simulink model "MCity_cs_withAEBSBlock"  (R2017a)
settings: Solver=ode5  StartTime=0.0  StopTime=3.95  FixedStep=1/200  RelTol=1e-3
PreLoadFcn:
  | check_NUTS_defined;
  | 
  | assignin('base',['model_closed_' bdroot],false);
InitFcn:
  | PreScanExperimentInitFcn(bdroot)
StopFcn:
  | PreScanExperimentStopFcn(bdroot)
model workspace (MAT data in the model file):
  mbox_table : struct (value not decoded)
  model_closed = 0
  sim_status = 0
values from neighbouring files (symbols this model uses):
  d_offset = -18.15    [monocityTestLeftTurn.mat]    (also in simulation_leftTurn_PreScan.m = dl/vl*vh - 43 + R)
undefined symbols (not defined in the file or in its folder): DiscIntNeverNeededParam, warningInitialVelocity, x0
libraries: simulink x78, PreScanSimulinkLibrary x14, simulink_extras x10, PreScanUsefulBlocks x4
(part 11 of 12)

== system MCity_cs_withAEBSBlock/BMW_Z3_1/Subsystem/PreBraking Model/Straight road segment/Impact point2 ==
  note: === Impact point block ===
      |
      |    - determines predicted distance to the point of impact,
      |    - passing through zero value, if there is no risk of collision.
  alfa : Inport
  xp [m] : Inport  Port=2
  yp [m] : Inport  Port=3
  Abs : Abs
  Add : Sum  Inputs=+-
  Compare To Constant : simulink/Logic and Bit Operations/Compare To Constant  relop=<  const=-1e-6  OutDataTypeStr=uint8  ZeroCross=off
  Compare To Constant1 : simulink/Logic and Bit Operations/Compare To Constant  relop=>  const=1e-6  OutDataTypeStr=uint8  ZeroCross=off
  Constant : Constant  Value=0
  Divide : Product  Inputs=*/
  Logical Operator : Logic  Operator=OR  AllPortsSameDT=off  OutDataTypeStr=boolean
  Saturation : Saturate  UpperLimit=inf  LowerLimit=1e-6
  Saturation1 : Saturate  UpperLimit=-1e-6  LowerLimit=-inf
  Saturation2 : Saturate  UpperLimit=300  LowerLimit=0
  Switch : Switch  Criteria=u2 > Threshold  Threshold=LaneWidth/2
  Switch1 : Switch  Criteria=u2 > Threshold  Threshold=0.5
  Switch2 : Switch  Criteria=u2 > Threshold
  Trigonometric Function : Trigonometry  Operator=tan
  xp [m]1 : InportShadow  Port=2
  yp [m]1 : InportShadow  Port=3
  xc [m] : Outport
  wires:
  yp [m]/1 -> Abs/1
  xp [m]/1 -> Switch/3
  Constant/1 -> Switch/1
  Switch/1 -> Switch1/3
  Abs/1 -> Switch/2
  xp [m]1/1 -> Add/1
  Divide/1 -> Add/2
  yp [m]1/1 -> Divide/1
  Trigonometric Function/1 -> Divide/2
  alfa/1 -> Compare To Constant1/1, Compare To Constant/1, Saturation1/1, Switch2/2, Saturation/1
  Compare To Constant1/1 -> Logical Operator/1
  Compare To Constant/1 -> Logical Operator/2
  Logical Operator/1 -> Switch1/2
  Switch1/1 -> Saturation2/1
  Add/1 -> Switch1/1
  Switch2/1 -> Trigonometric Function/1
  Saturation/1 -> Switch2/1
  Saturation1/1 -> Switch2/3
  Saturation2/1 -> xc [m]/1

== system MCity_cs_withAEBSBlock/BMW_Z3_1/Subsystem/PreBraking Model/Straight road segment/Relative velocity1 ==
  note: === Relative velocity block ===
      |
      |    - determines:
      |      -- relative, carthesian position of an obstacle,
      |      -- absolute values of carthesian velocity of an obstacle
      |          in respect to the actor orientation,
      |      -- relative velocity Vw beetwen actor and an obstacle
      |          in respect to actor front direction (x).
  V [m/s] : Inport
  range [m] : Inport  Port=2
  rangedot [m/s] : Inport  Port=3
  theta [rad] : Inport  Port=4
  theta_p [rad/s] : Inport  Port=5
  Abs{,1..3} (4 alike) : Abs
  Add : Sum  Inputs=++-
  Add2 : Sum  Inputs=-+
  Constant{,1..3} (4 alike) : Constant  Value=0
  Difference : simulink/Discrete/Difference  ICPrevInput=zeros(TISdet(1),1)  InputProcessing=Inherited  OutMin=[]  OutMax=[]  OutDataType=fixdt(1, 16)  OutScaling=2^-10  DoSatur=off
  Difference1 : simulink/Discrete/Difference  ICPrevInput=zeros(TISdet(1),1)  InputProcessing=Inherited  OutMin=[]  OutMax=[]  OutDataType=fixdt(1, 16)  OutScaling=2^-10  DoSatur=off
  Difference2 : simulink/Discrete/Difference  ICPrevInput=0.0  InputProcessing=Inherited  OutMin=[]  OutMax=[]  OutDataType=sfix(16)  OutScaling=2^-10  DoSatur=off
  Divide : Product  Inputs=**
  Divide1 : Product  Inputs=***
  Divide4 : Product  Inputs=**
  Divide6 : Product  Inputs=**
  Embedded MATLAB Function1 : MATLAB Function  TreatAsAtomicUnit=on
  Gain : Gain  Gain=0.01
  Saturation1 : Saturate  UpperLimit=50  LowerLimit=-50
  Saturation2 : Saturate  UpperLimit=150  LowerLimit=0
  Saturation3 : Saturate  UpperLimit=50  LowerLimit=-50
  Saturation4 : Saturate  UpperLimit=50  LowerLimit=-50
  Saturation5 : Saturate  UpperLimit=11.8  LowerLimit=-11.8
  Switch : Switch  Threshold=0.5
  Switch1 : Switch  Criteria=u2 > Threshold  Threshold=0.8
  Switch2 : Switch  Threshold=10
  Switch3 : Switch  Criteria=u2 > Threshold  Threshold=10
  Translation : MATLAB Function  TreatAsAtomicUnit=on
  Unit Delay : UnitDelay  InitialCondition=zeros(TISdet(1),50)  SampleTime=-1
  cos_theta : Trigonometry  Operator=cos
  sin_theta : Trigonometry
  yp' [m/s] : Outport
  xp' [m/s] : Outport  Port=2
  xp [m] : Outport  Port=3
  yp [m] : Outport  Port=4
  Vw [m/s] : Outport  Port=5
  wires:
  theta [rad]/1 -> cos_theta/1, sin_theta/1
  Divide/1 -> Saturation2/1
  range [m]/1 -> Divide/2, Divide6/1, Divide1/1, Embedded MATLAB Function1/1(r)
  sin_theta/1 -> Divide6/2, Divide1/2
  cos_theta/1 -> Divide/1, Divide4/1
  Divide6/1 -> Saturation5/1
  theta_p [rad/s]/1 -> Divide1/3
  Add2/1 -> Saturation3/1
  Divide4/1 -> Add2/1, Add/2
  Divide1/1 -> Add2/2, Add/3
  Saturation2/1 -> xp [m]/1
  Saturation5/1 -> Embedded MATLAB Function1/2(yp1), yp [m]/1
  Saturation1/1 -> Abs/1, Switch/1
  V [m/s]/1 -> Translation/1(v), Add/1
  Add/1 -> Saturation1/1
  Abs/1 -> Switch/2
  Constant/1 -> Switch/3
  Switch/1 -> Translation/2(xpd)
  Embedded MATLAB Function1/2(K2) -> Unit Delay/1
  Unit Delay/1 -> Embedded MATLAB Function1/3(K1)
  Embedded MATLAB Function1/1(yp2) -> Difference2/1
  Difference2/1 -> Gain/1
  Abs1/1 -> Switch1/2
  Constant1/1 -> Switch1/3
  Saturation4/1 -> yp' [m/s]/1
  Switch1/1 -> Difference/1, Switch2/3
  Switch2/1 -> Saturation4/1
  Difference/1 -> Abs2/1
  Abs2/1 -> Switch2/2
  Translation/1(xp_dot) -> Switch3/3, Difference1/1
  Abs3/1 -> Switch3/2
  Switch3/1 -> xp' [m/s]/1
  Constant2/1 -> Switch2/1
  Constant3/1 -> Switch3/1
  Difference1/1 -> Abs3/1
  rangedot [m/s]/1 -> Divide4/2
  Gain/1 -> Abs1/1, Switch1/1
  Saturation3/1 -> Vw [m/s]/1

== system MCity_cs_withAEBSBlock/BMW_Z3_1/Subsystem/PreBraking Model/Straight road segment/Relative velocity2 ==
  note: === Relative velocity block ===
      |
      |    - determines:
      |      -- relative, carthesian position of an obstacle,
      |      -- absolute values of carthesian velocity of an obstacle
      |          in respect to the actor orientation,
      |      -- relative velocity Vw beetwen actor and an obstacle
      |          in respect to actor front direction (x).
  V [m/s] : Inport
  range [m] : Inport  Port=2
  rangedot [m/s] : Inport  Port=3
  theta [rad] : Inport  Port=4
  theta_p [rad/s] : Inport  Port=5
  Abs{,1..3} (4 alike) : Abs
  Add : Sum  Inputs=++-
  Add2 : Sum  Inputs=-+
  Constant{,1..3} (4 alike) : Constant  Value=0
  Difference : simulink/Discrete/Difference  ICPrevInput=zeros(TISdet(2),1)  InputProcessing=Inherited  OutMin=[]  OutMax=[]  OutDataType=fixdt(1, 16)  OutScaling=2^-10  DoSatur=off
  Difference1 : simulink/Discrete/Difference  ICPrevInput=zeros(TISdet(2),1)  InputProcessing=Inherited  OutMin=[]  OutMax=[]  OutDataType=fixdt(1, 16)  OutScaling=2^-10  DoSatur=off
  Difference2 : simulink/Discrete/Difference  ICPrevInput=0.0  InputProcessing=Inherited  OutMin=[]  OutMax=[]  OutDataType=sfix(16)  OutScaling=2^-10  DoSatur=off
  Divide : Product  Inputs=**
  Divide1 : Product  Inputs=***
  Divide4 : Product  Inputs=**
  Divide6 : Product  Inputs=**
  Embedded MATLAB Function1 : MATLAB Function  TreatAsAtomicUnit=on  SystemSampleTime=0.01
  Gain : Gain  Gain=0.01
  Saturation1 : Saturate  UpperLimit=50  LowerLimit=-50
  Saturation2 : Saturate  UpperLimit=150  LowerLimit=0
  Saturation3 : Saturate  UpperLimit=50  LowerLimit=-50
  Saturation4 : Saturate  UpperLimit=50  LowerLimit=-50
  Saturation5 : Saturate  UpperLimit=11.8  LowerLimit=-11.8
  Switch : Switch  Threshold=0.5
  Switch1 : Switch  Criteria=u2 > Threshold  Threshold=0.8
  Switch2 : Switch  Threshold=10
  Switch3 : Switch  Criteria=u2 > Threshold  Threshold=10
  Translation : MATLAB Function  TreatAsAtomicUnit=on
  Unit Delay : UnitDelay  InitialCondition=zeros(TISdet(2),50)  SampleTime=-1
  cos_theta : Trigonometry  Operator=cos
  sin_theta : Trigonometry
  yp' [m/s] : Outport
  xp' [m/s] : Outport  Port=2
  xp [m] : Outport  Port=3
  yp [m] : Outport  Port=4
  Vw [m/s] : Outport  Port=5
  wires:
  rangedot [m/s]/1 -> Divide4/2
  Difference1/1 -> Abs3/1
  Constant3/1 -> Switch3/1
  Constant2/1 -> Switch2/1
  Switch3/1 -> xp' [m/s]/1
  Abs3/1 -> Switch3/2
  Translation/1(xp_dot) -> Difference1/1, Switch3/3
  Abs2/1 -> Switch2/2
  Difference/1 -> Abs2/1
  Switch2/1 -> Saturation4/1
  Switch1/1 -> Switch2/3, Difference/1
  Saturation4/1 -> yp' [m/s]/1
  Constant1/1 -> Switch1/3
  Abs1/1 -> Switch1/2
  Gain/1 -> Switch1/1, Abs1/1
  Embedded MATLAB Function1/1(yp2) -> Difference2/1
  Unit Delay/1 -> Embedded MATLAB Function1/3(K1)
  Embedded MATLAB Function1/2(K2) -> Unit Delay/1
  Switch/1 -> Translation/2(xpd)
  Constant/1 -> Switch/3
  Abs/1 -> Switch/2
  Add/1 -> Saturation1/1
  V [m/s]/1 -> Translation/1(v), Add/1
  Saturation1/1 -> Switch/1, Abs/1
  Saturation5/1 -> yp [m]/1, Embedded MATLAB Function1/2(yp1)
  Saturation2/1 -> xp [m]/1
  Divide1/1 -> Add/3, Add2/2
  Divide4/1 -> Add/2, Add2/1
  Add2/1 -> Saturation3/1
  theta_p [rad/s]/1 -> Divide1/3
  Divide6/1 -> Saturation5/1
  cos_theta/1 -> Divide/1, Divide4/1
  sin_theta/1 -> Divide6/2, Divide1/2
  range [m]/1 -> Embedded MATLAB Function1/1(r), Divide1/1, Divide6/1, Divide/2
  Divide/1 -> Saturation2/1
  theta [rad]/1 -> cos_theta/1, sin_theta/1
  Difference2/1 -> Gain/1
  Saturation3/1 -> Vw [m/s]/1

== system MCity_cs_withAEBSBlock/BMW_Z3_1/Subsystem/PreBraking Model/Straight road segment/T0.6 ==
  note: === T1.6 block ==
      |
      |    - compare TTC and output adequate binary flag.
  TTC : Inport
  Constant TTC : Inport  Port=2
  Gain : Gain  Gain=2
  Gain2 : Gain  Gain=ones(TISdet(2),1)
  Relational Operator1 : RelationalOperator  Operator=<  OutDataTypeStr=fixdt(1,16)  RndMeth=Nearest
  Switch : Switch  Criteria=u2 > Threshold
  all_flags_0,6 : Outport
  wires:
  Switch/1 -> Relational Operator1/1
  TTC/1 -> Switch/2, Switch/1
  Constant TTC/1 -> Gain2/1
  Gain/1 -> Switch/3
  Gain2/1 -> Gain/1, Relational Operator1/2
  Relational Operator1/1 -> all_flags_0,6/1

== system MCity_cs_withAEBSBlock/BMW_Z3_1/Subsystem/PreBraking Model/Straight road segment/T1.6 ==
  note: === T1.6 block ==
      |
      |    - compare TTC and output adequate binary flag.
  TTC : Inport
  Constant TTC : Inport  Port=2
  Gain : Gain  Gain=2
  Gain2 : Gain  Gain=ones(TISdet(1),1)
  Relational Operator1 : RelationalOperator  Operator=<  OutDataTypeStr=fixdt(1,16)  RndMeth=Nearest
  Switch : Switch  Criteria=u2 > Threshold
  median filter : Subsystem
  all_flags_1.6 : Outport
  wires:
  Switch/1 -> Relational Operator1/1
  Relational Operator1/1 -> median filter/1(Flag in)
  TTC/1 -> Switch/2, Switch/1
  Constant TTC/1 -> Gain2/1
  Gain/1 -> Switch/3
  Gain2/1 -> Gain/1, Relational Operator1/2
  median filter/1(Flag out) -> all_flags_1.6/1

== system MCity_cs_withAEBSBlock/BMW_Z3_1/Subsystem/PreBraking Model/Straight road segment/T2.6 ==
  note: === T1.6 block ==
      |
      |    - compare TTC and output adequate binary flag.
  TTC : Inport
  Constant TTC : Inport  Port=2
  Gain : Gain  Gain=2
  Gain2 : Gain  Gain=ones(TISdet(1),1)
  Relational Operator1 : RelationalOperator  Operator=<  OutDataTypeStr=fixdt(1,16)  RndMeth=Nearest
  Switch : Switch  Criteria=u2 > Threshold
  median filter : Subsystem
  all_flags_2.6 : Outport
  wires:
  Switch/1 -> Relational Operator1/1
  TTC/1 -> Switch/2, Switch/1
  Constant TTC/1 -> Gain2/1
  Gain/1 -> Switch/3
  Gain2/1 -> Gain/1, Relational Operator1/2
  Relational Operator1/1 -> median filter/1(Flag in)
  median filter/1(Flag out) -> all_flags_2.6/1

== system MCity_cs_withAEBSBlock/BMW_Z3_1/Subsystem/PreBraking Model/Straight road segment/THETA Derivative1 ==
  note: === Theta derivative block ===
      |
      |    - computs derivative of the theta using linear
      |       extrapolation and correction method
  range [m] : Inport
  theta [rad] : Inport  Port=2
  Abs1 : Abs
  Deriv correction : MATLAB Function  TreatAsAtomicUnit=on
  Difference1 : simulink/Discrete/Difference  ICPrevInput=0.0  InputProcessing=Inherited  OutMin=[]  OutMax=[]  OutDataType=sfix(16)  OutScaling=2^-10  DoSatur=off
  Difference2 : simulink/Discrete/Difference  ICPrevInput=0.0  InputProcessing=Inherited  OutMin=[]  OutMax=[]  OutDataType=sfix(16)  OutScaling=2^-10  DoSatur=off
  Digital Clock : DigitalClock  SampleTime=min(Tsensor)
  Gain : Gain  Gain=Tsensor(2)
  Gain1 : Gain  Gain=Tsensor(2)
  Switch : Switch  Threshold=2
  Theta extrapolation : MATLAB Function  TreatAsAtomicUnit=on
  Unit Delay : UnitDelay  InitialCondition=zeros(TISdet(2),1)  SampleTime=-1
  Unit Delay1 : UnitDelay  InitialCondition=zeros(TISdet(2),10,2)  SampleTime=-1
  Unit Delay2 : UnitDelay  InitialCondition=zeros(TISdet(2),1)  SampleTime=-1
  theta_dot [rad/s] : Outport
  wires:
  Unit Delay2/1 -> Deriv correction/2(thp)
  Gain1/1 -> Deriv correction/3(thd)
  Theta extrapolation/1(th2) -> Deriv correction/1(th), Unit Delay2/1, Difference1/1
  range [m]/1 -> Theta extrapolation/1(r)
  Gain/1 -> Theta extrapolation/3(thd)
  Digital Clock/1 -> Theta extrapolation/4(time)
  Unit Delay1/1 -> Theta extrapolation/5(K1)
  Theta extrapolation/2(K2) -> Unit Delay1/1
  theta [rad]/1 -> Theta extrapolation/2(th1), Difference2/1
  Deriv correction/1(th_dot) -> Switch/3, Abs1/1
  Switch/1 -> theta_dot [rad/s]/1, Unit Delay/1
  Abs1/1 -> Switch/2
  Unit Delay/1 -> Switch/1
  Difference2/1 -> Gain/1
  Difference1/1 -> Gain1/1

== system MCity_cs_withAEBSBlock/BMW_Z3_1/Subsystem/PreBraking Model/Straight road segment/THETA Derivative2 ==
  note: === Theta derivative block ===
      |
      |    - computs derivative of the theta using linear
      |       extrapolation and correction method
  range [m] : Inport
  theta [rad] : Inport  Port=2
  Abs1 : Abs
  Deriv correction : MATLAB Function  TreatAsAtomicUnit=on
  Difference1 : simulink/Discrete/Difference  ICPrevInput=0.0  InputProcessing=Inherited  OutMin=[]  OutMax=[]  OutDataType=sfix(16)  OutScaling=2^-10  DoSatur=off
  Difference2 : simulink/Discrete/Difference  ICPrevInput=0.0  InputProcessing=Inherited  OutMin=[]  OutMax=[]  OutDataType=sfix(16)  OutScaling=2^-10  DoSatur=off
  Digital Clock : DigitalClock  SampleTime=min(Tsensor)
  Gain : Gain  Gain=Tsensor(1)
  Gain1 : Gain  Gain=Tsensor(1)
  Switch : Switch  Threshold=2
  Theta extrapolation : MATLAB Function  TreatAsAtomicUnit=on
  Unit Delay : UnitDelay  InitialCondition=zeros(TISdet(1),1)  SampleTime=-1
  Unit Delay1 : UnitDelay  InitialCondition=zeros(TISdet(1),10,2)  SampleTime=-1
  Unit Delay2 : UnitDelay  InitialCondition=zeros(TISdet(1),1)  SampleTime=-1
  theta_dot [rad/s] : Outport
  wires:
  Unit Delay2/1 -> Deriv correction/2(thp)
  Gain1/1 -> Deriv correction/3(thd)
  Theta extrapolation/1(th2) -> Deriv correction/1(th), Unit Delay2/1, Difference1/1
  range [m]/1 -> Theta extrapolation/1(r)
  Gain/1 -> Theta extrapolation/3(thd)
  Digital Clock/1 -> Theta extrapolation/4(time)
  Unit Delay1/1 -> Theta extrapolation/5(K1)
  Theta extrapolation/2(K2) -> Unit Delay1/1
  theta [rad]/1 -> Theta extrapolation/2(th1), Difference2/1
  Deriv correction/1(th_dot) -> Switch/3, Abs1/1
  Switch/1 -> theta_dot [rad/s]/1, Unit Delay/1
  Abs1/1 -> Switch/2
  Unit Delay/1 -> Switch/1
  Difference2/1 -> Gain/1
  Difference1/1 -> Gain1/1

== system MCity_cs_withAEBSBlock/BMW_Z3_1/Subsystem/PreBraking Model/Straight road segment/TTC computing ==
  xc [m] : Inport
  Vw [m/s] : Inport  Port=2
  Compare To Constant : simulink/Logic and Bit Operations/Compare To Constant  relop===  const=1e-6  OutDataTypeStr=uint8  ZeroCross=off
  Constant : Constant  Value=0
  Data Type Conversion : DataTypeConversion
  Divide : Product  Inputs=/*
  Saturation : Saturate  UpperLimit=inf  LowerLimit=1e-6
  Switch : Switch  Criteria=u2 > Threshold
  Switch1 : Switch  Criteria=u2 > Threshold  Threshold=0.5
  TTC : Outport  InitialOutput=0
  wires:
  Vw [m/s]/1 -> Switch/2, Switch/1
  Constant/1 -> Switch1/1, Switch/3
  Switch/1 -> Saturation/1
  Saturation/1 -> Divide/1, Compare To Constant/1
  Compare To Constant/1 -> Data Type Conversion/1
  xc [m]/1 -> Divide/2
  Divide/1 -> Switch1/3
  Switch1/1 -> TTC/1
  Data Type Conversion/1 -> Switch1/2

== system MCity_cs_withAEBSBlock/BMW_Z3_1/Subsystem/PreBraking Model/Straight road segment/TTC computing1 ==
  xc [m] : Inport
  Vw [m/s] : Inport  Port=2
  Compare To Constant : simulink/Logic and Bit Operations/Compare To Constant  relop===  const=1e-6  OutDataTypeStr=uint8  ZeroCross=off
  Constant : Constant  Value=0
  Data Type Conversion : DataTypeConversion
  Divide : Product  Inputs=/*
  Saturation : Saturate  UpperLimit=inf  LowerLimit=1e-6
  Switch : Switch  Criteria=u2 > Threshold
  Switch1 : Switch  Criteria=u2 > Threshold  Threshold=0.5
  TTC : Outport  InitialOutput=0
  wires:
  Vw [m/s]/1 -> Switch/2, Switch/1
  Constant/1 -> Switch/3, Switch1/1
  Switch/1 -> Saturation/1
  Saturation/1 -> Divide/1, Compare To Constant/1
  Compare To Constant/1 -> Data Type Conversion/1
  xc [m]/1 -> Divide/2
  Divide/1 -> Switch1/3
  Switch1/1 -> TTC/1
  Data Type Conversion/1 -> Switch1/2

== system MCity_cs_withAEBSBlock/BMW_Z3_1/Subsystem/PreBraking Model/Straight road segment/alfa ==
  yp'1 : Inport
  xp' : Inport  Port=2
  Abs : Abs
  Compare To Constant : simulink/Logic and Bit Operations/Compare To Constant  relop===  const=pi/2  OutDataTypeStr=uint8
  Constant : Constant  Value=0
  Switch : Switch  Criteria=u2 > Threshold
  four quadrant atan : Trigonometry  Operator=atan2
  alfa1 : Outport
  wires:
  yp'1/1 -> four quadrant atan/1
  xp'/1 -> four quadrant atan/2
  four quadrant atan/1 -> Abs/1, Switch/3
  Abs/1 -> Compare To Constant/1
  Compare To Constant/1 -> Switch/2
  Constant/1 -> Switch/1
  Switch/1 -> alfa1/1

== system MCity_cs_withAEBSBlock/BMW_Z3_1/Subsystem/PreBraking Model/Straight road segment/alfa1 ==
  yp'1 : Inport
  xp' : Inport  Port=2
  Abs : Abs
  Compare To Constant : simulink/Logic and Bit Operations/Compare To Constant  relop===  const=pi/2  OutDataTypeStr=uint8
  Constant : Constant  Value=0
  Switch : Switch  Criteria=u2 > Threshold
  four quadrant atan : Trigonometry  Operator=atan2
  alfa1 : Outport
  wires:
  yp'1/1 -> four quadrant atan/1
  xp'/1 -> four quadrant atan/2
  four quadrant atan/1 -> Abs/1, Switch/3
  Abs/1 -> Compare To Constant/1
  Compare To Constant/1 -> Switch/2
  Constant/1 -> Switch/1
  Switch/1 -> alfa1/1

== system MCity_cs_withAEBSBlock/BMW_Z3_1/Trajectories/Traj2State1/Traj2State2/MuxState ==
  x [m] : Inport
  y [m] : Inport  Port=2
  z [m] : Inport  Port=3
  dx [m/s] : Inport  Port=4
  dy [m/s] : Inport  Port=5
  dz [m/s] : Inport  Port=6
  R [rad] : Inport  Port=7
  P [rad] : Inport  Port=8
  Y [rad] : Inport  Port=9
  Mux : Mux  Inputs=9
  state : Outport
  wires:
  z [m]/1 -> Mux/3
  y [m]/1 -> Mux/2
  x [m]/1 -> Mux/1
  Y [rad]/1 -> Mux/9
  P [rad]/1 -> Mux/8
  R [rad]/1 -> Mux/7
  dz [m/s]/1 -> Mux/6
  dy [m/s]/1 -> Mux/5
  dx [m/s]/1 -> Mux/4
  Mux/1 -> state/1

== system MCity_cs_withAEBSBlock/BMW_Z3_1/Trajectories/Traj2State1/Traj2State2/Traj2MuxState_Ext ==
  Traj : Inport
  Terminator{1..9} (9 alike) : Terminator
  demux : Subsystem
  x [m] : Outport
  y [m] : Outport  Port=2
  z [m] : Outport  Port=3
  dx [m/s] : Outport  Port=4
  dy [m/s] : Outport  Port=5
  dz [m/s] : Outport  Port=6
  R [rad] : Outport  Port=7
  P [rad] : Outport  Port=8
  Y [rad] : Outport  Port=9
  wires:
  demux/9(Y) -> Y [rad]/1
  demux/7(R) -> R [rad]/1
  demux/5(vely) -> dy [m/s]/1
  demux/4(velx) -> dx [m/s]/1
  demux/10(velR) -> Terminator4/1
  demux/11(velP) -> Terminator5/1
  demux/12(velY) -> Terminator1/1
  demux/13(accx) -> Terminator8/1
  demux/14(accy) -> Terminator9/1
  demux/15(accz) -> Terminator7/1
  demux/18(accY) -> Terminator2/1
  demux/16(accR) -> Terminator3/1
  demux/17(accP) -> Terminator6/1
  demux/3(z) -> z [m]/1
  Traj/1 -> demux/1(traj)
  demux/6(velz) -> dz [m/s]/1
  demux/1(x) -> x [m]/1
  demux/2(y) -> y [m]/1
  demux/8(P) -> P [rad]/1

== system MCity_cs_withAEBSBlock/Audi_A8_1/Dynamics_Simple/Chassis/Bicycle_model_[XYZ]/X_Motion/Air&RoadResistance ==
  vx_[ms-1] : Inport
  Gain : Gain  Gain=1/p.Rw
  Road & Aerodyn Resistances : Fcn  Expr=p.Rroad + p.Rair*u^2
  Saturation1 : Saturate  UpperLimit=5/15  LowerLimit=-5/15
  Sign : Signum
  "[ms-1] 2 [rads-1]" : Gain  Gain=1/p.Rw  SaturateOnIntegerOverflow=on  OutDataTypeStr=Inherit: Same as input  ParamDataTypeStr=Inherit: Same as input
  signed load1 : Product  SaturateOnIntegerOverflow=on  InputSameDT=on  OutDataTypeStr=Inherit: Same as first input
  Resistance_Force : Outport
  wires:
  signed load1/1 -> Resistance_Force/1  "F_[N]"
  vx_[ms-1]/1 -> Road & Aerodyn Resistances/1, "[ms-1] 2 [rads-1]"/1
  Saturation1/1 -> Sign/1
  "[ms-1] 2 [rads-1]"/1 -> Saturation1/1
  Road & Aerodyn Resistances/1 -> Gain/1  "ResistanceTorque_[Nm]"
  Sign/1 -> signed load1/2  "sign"
  Gain/1 -> signed load1/1  "Resistance Force_[N]"

== system MCity_cs_withAEBSBlock/Audi_A8_1/Dynamics_Simple/Chassis/Bicycle_model_[XYZ]/X_Motion/BrakeSystem ==
  vx_[ms-1] : Inport
  BrakePressure_[bar] : Inport  Port=2
  Gain : Gain  Gain=1/p.Rw
  Saturation : Saturate  UpperLimit=p.PBrakeMax  LowerLimit=0
  Saturation1 : Saturate  UpperLimit=5/15  LowerLimit=-5/15
  Sign : Signum
  "[ms-1] 2 [rads-1]" : Gain  Gain=1/p.Rw  SaturateOnIntegerOverflow=on  OutDataTypeStr=Inherit: Same as input  ParamDataTypeStr=Inherit: Same as input
  braking Q factor : Gain  Gain=p.Qfac  SaturateOnIntegerOverflow=on  OutDataTypeStr=Inherit: Same as input  ParamDataTypeStr=Inherit: Same as input
  signed load1 : Product  SaturateOnIntegerOverflow=on  InputSameDT=on  OutDataTypeStr=Inherit: Same as first input
  BrakeForce : Outport
  BrakeTorqueAbs : Outport  Port=2
  wires:
  braking Q factor/1 -> BrakeTorqueAbs/1, Gain/1
  BrakePressure_[bar]/1 -> Saturation/1
  Saturation/1 -> braking Q factor/1
  vx_[ms-1]/1 -> "[ms-1] 2 [rads-1]"/1
  Saturation1/1 -> Sign/1
  "[ms-1] 2 [rads-1]"/1 -> Saturation1/1
  Sign/1 -> signed load1/2  "sign"
  signed load1/1 -> BrakeForce/1
  Gain/1 -> signed load1/1

== system MCity_cs_withAEBSBlock/Audi_A8_1/Dynamics_Simple/Chassis/Bicycle_model_[XYZ]/X_Motion/Configurable Subsystem ==
  In1 : Inport
  In2 : Inport  Port=2
  In3 : Inport  Port=3
  Integrator : Integrator  ExternalReset=level  InitialConditionSource=external
  Out1 : Outport
  wires:
  In1/1 -> Integrator/1
  In2/1 -> Integrator/2
  In3/1 -> Integrator/3
  Integrator/1 -> Out1/1

== system MCity_cs_withAEBSBlock/Audi_A8_1/Dynamics_Simple/Chassis/Bicycle_model_[XYZ]/X_Motion/Configurable Subsystem1 ==
  In1 : Inport
  Torsional damping : TransferFcn  Denominator=[0.1 1]
  Out1 : Outport
  wires:
  In1/1 -> Torsional damping/1
  Torsional damping/1 -> Out1/1

== system MCity_cs_withAEBSBlock/Audi_A8_1/Dynamics_Simple/Chassis/Bicycle_model_[XYZ]/X_Motion/Max RPM and zero- velocity detection ==
  note: Set to zero after infinite small time-step
  note: Zero velocity detection
  ax : Inport
  Drive Torque : Inport  Port=2
  Brake Torque : Inport  Port=3
  v0 : Inport  Port=4
  vx : Inport  Port=5
  Abs : Abs
  Abs1 : Abs
  Compare To Zero : simulink/Logic and Bit Operations/Compare To Zero  relop=<=  OutDataTypeStr=boolean  ZeroCross=off
  Compare To Zero1 : simulink/Logic and Bit Operations/Compare To Zero  relop=>=  OutDataTypeStr=boolean  ZeroCross=off
  Compare To Zero2 : simulink/Logic and Bit Operations/Compare To Zero  relop=>=  OutDataTypeStr=boolean  ZeroCross=off
  Compare To Zero3 : simulink/Logic and Bit Operations/Compare To Zero  relop=<=  OutDataTypeStr=boolean  ZeroCross=off
  Configurable Subsystem : Subsystem  BlockChoice=Step  mask{ComputationMode=ComputationMode}
      mask prompts: ComputationMode "Compuation mode:"
      mask init:
      | SetComputationMode(gcb,ComputationMode);
      settings: AttributesFormatString=%<BlockChoice>  OpenFcn=BringToFront(gcb);  MemberBlocks=Discrete Step,Step
      settings: TemplateBlock=|
      | PreScanSimulinkLibrary/Configurable Subsystems/Step Function/Configurable
      | Subsystem
  Constant : Constant
  Constant1 : Constant
  Logical Operator : Logic  AllPortsSameDT=off  OutDataTypeStr=boolean
  Logical Operator1 : Logic  AllPortsSameDT=off  OutDataTypeStr=boolean
  Logical Operator2 : Logic  Operator=NOT  AllPortsSameDT=off  OutDataTypeStr=boolean
  Logical Operator3 : Logic  AllPortsSameDT=off  OutDataTypeStr=boolean
  Logical Operator4 : Logic  Operator=OR  AllPortsSameDT=off  OutDataTypeStr=boolean
  Memory : Memory
  Memory1 : Memory
  Memory2 : Memory
  Product : Product  RndMeth=Zero
  Relational Operator : RelationalOperator  Operator=<  OutDataTypeStr=boolean  RndMeth=Nearest
  SR-Memory : Subsystem
  Sum : Sum  Inputs=|-+
  Switch : Switch  Criteria=u2 ~= 0  Threshold=0.5
  ax is 0 : Constant  Value=0
  ax_out : Outport
  vx_reset : Outport  Port=2
  x0 : Outport  Port=3
  wires:
  Logical Operator4/1 -> Logical Operator1/1
  vx/1 -> Compare To Zero/1, Compare To Zero2/1, Memory2/1, Memory/1  "vx"
  Memory2/1 -> Compare To Zero3/1
  Compare To Zero2/1 -> Logical Operator3/1
  Compare To Zero3/1 -> Logical Operator3/2
  Logical Operator3/1 -> Logical Operator4/2  "zero-crossing backward"
  Memory/1 -> Compare To Zero1/1
  Compare To Zero/1 -> Logical Operator/1
  Compare To Zero1/1 -> Logical Operator/2
  Logical Operator/1 -> Logical Operator4/1  "zero-crossing forward"
  Abs/1 -> Relational Operator/1
  Abs1/1 -> Relational Operator/2
  Drive Torque/1 -> Abs/1
  Brake Torque/1 -> Abs1/1
  Relational Operator/1 -> Logical Operator1/2, Logical Operator2/1
  Logical Operator1/1 -> SR-Memory/2(Set)
  Constant/1 -> SR-Memory/1(Signal)
  Logical Operator2/1 -> SR-Memory/3(Reset)
  SR-Memory/1(Out) -> Sum/1, Memory1/1
  Switch/1 -> ax_out/1
  Sum/1 -> Switch/2
  ax is 0/1 -> Switch/3
  Constant1/1 -> Sum/2
  v0/1 -> Product/1
  Product/1 -> x0/1
  Configurable Subsystem/1(Out1) -> Product/2
  ax/1 -> Switch/1  "ax"
  Memory1/1 -> vx_reset/1  "vx"

== system MCity_cs_withAEBSBlock/Audi_A8_1/Dynamics_Simple/Chassis/Bicycle_model_[XYZ]/Y & Yaw_Motion/Configurable Subsystem ==
  In1 : Inport
  In2 : Inport  Port=2
  Integrator : Integrator  ExternalReset=level
  Out1 : Outport
  wires:
  In1/1 -> Integrator/1
  In2/1 -> Integrator/2
  Integrator/1 -> Out1/1

== system MCity_cs_withAEBSBlock/Audi_A8_1/Dynamics_Simple/Chassis/Bicycle_model_[XYZ]/Y & Yaw_Motion/Configurable Subsystem1 ==
  In1 : Inport
  Integrator : Integrator
  Out1 : Outport
  wires:
  In1/1 -> Integrator/1
  Integrator/1 -> Out1/1

== system MCity_cs_withAEBSBlock/Audi_A8_1/Dynamics_Simple/Chassis/Bicycle_model_[XYZ]/Y & Yaw_Motion/Configurable Subsystem2 ==
  In1 : Inport
  In2 : Inport  Port=2
  Integrator : Integrator  ExternalReset=level
  Out1 : Outport
  wires:
  In1/1 -> Integrator/1
  In2/1 -> Integrator/2
  Integrator/1 -> Out1/1

== system MCity_cs_withAEBSBlock/Audi_A8_1/Dynamics_Simple/Chassis/Bicycle_model_[XYZ]/Z, Pitch_Motion & Roll_Motion/Configurable Subsystem ==
  In1 : Inport
  Integrator : Integrator  LimitOutput=on  UpperSaturationLimit=5*pi/180  LowerSaturationLimit=-5*pi/180
  Out1 : Outport
  wires:
  In1/1 -> Integrator/1
  Integrator/1 -> Out1/1

== system MCity_cs_withAEBSBlock/Audi_A8_1/Dynamics_Simple/Chassis/Bicycle_model_[XYZ]/Z, Pitch_Motion & Roll_Motion/Configurable Subsystem1 ==
  In1 : Inport
  Integrator : Integrator
  Out1 : Outport
  wires:
  In1/1 -> Integrator/1
  Integrator/1 -> Out1/1

== system MCity_cs_withAEBSBlock/Audi_A8_1/Dynamics_Simple/Chassis/Bicycle_model_[XYZ]/Z, Pitch_Motion & Roll_Motion/Configurable Subsystem2 ==
  In1 : Inport
  Integrator : Integrator
  Out1 : Outport
  wires:
  In1/1 -> Integrator/1
  Integrator/1 -> Out1/1

== system MCity_cs_withAEBSBlock/Audi_A8_1/Dynamics_Simple/Chassis/Bicycle_model_[XYZ]/Z, Pitch_Motion & Roll_Motion/Configurable Subsystem3 ==
  In1 : Inport
  Integrator : Integrator
  Out1 : Outport
  wires:
  In1/1 -> Integrator/1
  Integrator/1 -> Out1/1

== system MCity_cs_withAEBSBlock/Audi_A8_1/Dynamics_Simple/Chassis/Bicycle_model_[XYZ]/Z, Pitch_Motion & Roll_Motion/Configurable Subsystem4 ==
  In1 : Inport
  Integrator : Integrator
  Out1 : Outport
  wires:
  In1/1 -> Integrator/1
  Integrator/1 -> Out1/1

== system MCity_cs_withAEBSBlock/Audi_A8_1/Dynamics_Simple/Chassis/Bicycle_model_[XYZ]/Z, Pitch_Motion & Roll_Motion/Configurable Subsystem5 ==
  In1 : Inport
  Integrator : Integrator
  Out1 : Outport
  wires:
  In1/1 -> Integrator/1
  Integrator/1 -> Out1/1

== system MCity_cs_withAEBSBlock/Audi_A8_1/Dynamics_Simple/Chassis/Bicycle_model_[XYZ]/Z, Pitch_Motion & Roll_Motion/Configurable Subsystem9 ==
  In1 : Inport
  Derivative : Derivative
  Out1 : Outport
  wires:
  In1/1 -> Derivative/1
  Derivative/1 -> Out1/1

== system MCity_cs_withAEBSBlock/Audi_A8_1/Dynamics_Simple/Chassis/FrontTyre/AlphaFront/Enabled Subsystem ==
  In : Inport
  Enable : EnablePort  PropagateVarSize=During execution
  AlphaFront : Fcn  Expr=-atan( (u(2)+u(3)*p.a)/u(1) )
  Alpha : Outport  OutputWhenDisabled=reset  InitialOutput=[0]
  wires:
  AlphaFront/1 -> Alpha/1
  In/1 -> AlphaFront/1

== system MCity_cs_withAEBSBlock/Audi_A8_1/Dynamics_Simple/Chassis/RearTyre/AlphaRear/Enabled Subsystem ==
  In : Inport
  Enable : EnablePort  PropagateVarSize=During execution
  AlphaRear : Fcn  Expr=-atan( (u(2)-u(3)*p.b)/u(1) )
  Alpha : Outport  OutputWhenDisabled=reset  InitialOutput=[0]
  wires:
  AlphaRear/1 -> Alpha/1
  In/1 -> AlphaRear/1

== system MCity_cs_withAEBSBlock/Audi_A8_1/Trajectories/Traj2State1/Traj2State2/Traj2MuxState_Ext/demux ==
  traj : Inport
  Demux : Demux  Outputs=18
  x : Outport
  y : Outport  Port=2
  z : Outport  Port=3
  velx : Outport  Port=4
  vely : Outport  Port=5
  velz : Outport  Port=6
  R : Outport  Port=7
  P : Outport  Port=8
  Y : Outport  Port=9
  velR : Outport  Port=10
  velP : Outport  Port=11
  velY : Outport  Port=12
  accx : Outport  Port=13
  accy : Outport  Port=14
  accz : Outport  Port=15
  accR : Outport  Port=16
  accP : Outport  Port=17
  accY : Outport  Port=18
  wires:
  Demux/18 -> accY/1
  Demux/17 -> accP/1
  Demux/16 -> accR/1
  Demux/15 -> accz/1
  Demux/14 -> accy/1
  Demux/13 -> accx/1
  Demux/12 -> velY/1
  Demux/11 -> velP/1
  Demux/10 -> velR/1
  Demux/9 -> velz/1
  Demux/8 -> vely/1
  Demux/7 -> velx/1
  Demux/6 -> Y/1
  Demux/5 -> P/1
  traj/1 -> Demux/1
  Demux/4 -> R/1
  Demux/3 -> z/1
  Demux/2 -> y/1
  Demux/1 -> x/1

== system MCity_cs_withAEBSBlock/BMW_Z3_1/Dynamics_Simple/Chassis/Bicycle_model_[XYZ]/X_Motion/Air&RoadResistance ==
  vx_[ms-1] : Inport
  Gain : Gain  Gain=1/p.Rw
  Road & Aerodyn Resistances : Fcn  Expr=p.Rroad + p.Rair*u^2
  Saturation1 : Saturate  UpperLimit=5/15  LowerLimit=-5/15
  Sign : Signum
  "[ms-1] 2 [rads-1]" : Gain  Gain=1/p.Rw  SaturateOnIntegerOverflow=on  OutDataTypeStr=Inherit: Same as input  ParamDataTypeStr=Inherit: Same as input
  signed load1 : Product  SaturateOnIntegerOverflow=on  InputSameDT=on  OutDataTypeStr=Inherit: Same as first input
  Resistance_Force : Outport
  wires:
  signed load1/1 -> Resistance_Force/1  "F_[N]"
  vx_[ms-1]/1 -> Road & Aerodyn Resistances/1, "[ms-1] 2 [rads-1]"/1
  Saturation1/1 -> Sign/1
  "[ms-1] 2 [rads-1]"/1 -> Saturation1/1
  Road & Aerodyn Resistances/1 -> Gain/1  "ResistanceTorque_[Nm]"
  Sign/1 -> signed load1/2  "sign"
  Gain/1 -> signed load1/1  "Resistance Force_[N]"

== system MCity_cs_withAEBSBlock/BMW_Z3_1/Dynamics_Simple/Chassis/Bicycle_model_[XYZ]/X_Motion/BrakeSystem ==
  vx_[ms-1] : Inport
  BrakePressure_[bar] : Inport  Port=2
  Gain : Gain  Gain=1/p.Rw
  Saturation : Saturate  UpperLimit=p.PBrakeMax  LowerLimit=0
  Saturation1 : Saturate  UpperLimit=5/15  LowerLimit=-5/15
  Sign : Signum
  "[ms-1] 2 [rads-1]" : Gain  Gain=1/p.Rw  SaturateOnIntegerOverflow=on  OutDataTypeStr=Inherit: Same as input  ParamDataTypeStr=Inherit: Same as input
  braking Q factor : Gain  Gain=p.Qfac  SaturateOnIntegerOverflow=on  OutDataTypeStr=Inherit: Same as input  ParamDataTypeStr=Inherit: Same as input
  signed load1 : Product  SaturateOnIntegerOverflow=on  InputSameDT=on  OutDataTypeStr=Inherit: Same as first input
  BrakeForce : Outport
  BrakeTorqueAbs : Outport  Port=2
  wires:
  braking Q factor/1 -> BrakeTorqueAbs/1, Gain/1
  BrakePressure_[bar]/1 -> Saturation/1
  Saturation/1 -> braking Q factor/1
  vx_[ms-1]/1 -> "[ms-1] 2 [rads-1]"/1
  Saturation1/1 -> Sign/1
  "[ms-1] 2 [rads-1]"/1 -> Saturation1/1
  Sign/1 -> signed load1/2  "sign"
  signed load1/1 -> BrakeForce/1
  Gain/1 -> signed load1/1

== system MCity_cs_withAEBSBlock/BMW_Z3_1/Dynamics_Simple/Chassis/Bicycle_model_[XYZ]/X_Motion/Configurable Subsystem ==
  In1 : Inport
  In2 : Inport  Port=2
  In3 : Inport  Port=3
  Integrator : Integrator  ExternalReset=level  InitialConditionSource=external
  Out1 : Outport
  wires:
  In1/1 -> Integrator/1
  In2/1 -> Integrator/2
  In3/1 -> Integrator/3
  Integrator/1 -> Out1/1

== system MCity_cs_withAEBSBlock/BMW_Z3_1/Dynamics_Simple/Chassis/Bicycle_model_[XYZ]/X_Motion/Configurable Subsystem1 ==
  In1 : Inport
  Torsional damping : TransferFcn  Denominator=[0.1 1]
  Out1 : Outport
  wires:
  In1/1 -> Torsional damping/1
  Torsional damping/1 -> Out1/1

== system MCity_cs_withAEBSBlock/BMW_Z3_1/Dynamics_Simple/Chassis/Bicycle_model_[XYZ]/X_Motion/Max RPM and zero- velocity detection ==
  note: Set to zero after infinite small time-step
  note: Zero velocity detection
  ax : Inport
  Drive Torque : Inport  Port=2
  Brake Torque : Inport  Port=3
  v0 : Inport  Port=4
  vx : Inport  Port=5
  Abs : Abs
  Abs1 : Abs
  Compare To Zero : simulink/Logic and Bit Operations/Compare To Zero  relop=<=  OutDataTypeStr=boolean  ZeroCross=off
  Compare To Zero1 : simulink/Logic and Bit Operations/Compare To Zero  relop=>=  OutDataTypeStr=boolean  ZeroCross=off
  Compare To Zero2 : simulink/Logic and Bit Operations/Compare To Zero  relop=>=  OutDataTypeStr=boolean  ZeroCross=off
  Compare To Zero3 : simulink/Logic and Bit Operations/Compare To Zero  relop=<=  OutDataTypeStr=boolean  ZeroCross=off
  Configurable Subsystem : Subsystem  BlockChoice=Step  mask{ComputationMode=ComputationMode}
      mask prompts: ComputationMode "Compuation mode:"
      mask init:
      | SetComputationMode(gcb,ComputationMode);
      settings: AttributesFormatString=%<BlockChoice>  OpenFcn=BringToFront(gcb);  MemberBlocks=Discrete Step,Step
      settings: TemplateBlock=|
      | PreScanSimulinkLibrary/Configurable Subsystems/Step Function/Configurable
      | Subsystem
  Constant : Constant
  Constant1 : Constant
  Logical Operator : Logic  AllPortsSameDT=off  OutDataTypeStr=boolean
  Logical Operator1 : Logic  AllPortsSameDT=off  OutDataTypeStr=boolean
  Logical Operator2 : Logic  Operator=NOT  AllPortsSameDT=off  OutDataTypeStr=boolean
  Logical Operator3 : Logic  AllPortsSameDT=off  OutDataTypeStr=boolean
  Logical Operator4 : Logic  Operator=OR  AllPortsSameDT=off  OutDataTypeStr=boolean
  Memory : Memory
  Memory1 : Memory
  Memory2 : Memory
  Product : Product  RndMeth=Zero
  Relational Operator : RelationalOperator  Operator=<  OutDataTypeStr=boolean  RndMeth=Nearest
  SR-Memory : Subsystem
  Sum : Sum  Inputs=|-+
  Switch : Switch  Criteria=u2 ~= 0  Threshold=0.5
  ax is 0 : Constant  Value=0
  ax_out : Outport
  vx_reset : Outport  Port=2
  x0 : Outport  Port=3
  wires:
  Logical Operator4/1 -> Logical Operator1/1
  vx/1 -> Compare To Zero/1, Compare To Zero2/1, Memory2/1, Memory/1  "vx"
  Memory2/1 -> Compare To Zero3/1
  Compare To Zero2/1 -> Logical Operator3/1
  Compare To Zero3/1 -> Logical Operator3/2
  Logical Operator3/1 -> Logical Operator4/2  "zero-crossing backward"
  Memory/1 -> Compare To Zero1/1
  Compare To Zero/1 -> Logical Operator/1
  Compare To Zero1/1 -> Logical Operator/2
  Logical Operator/1 -> Logical Operator4/1  "zero-crossing forward"
  Abs/1 -> Relational Operator/1
  Abs1/1 -> Relational Operator/2
  Drive Torque/1 -> Abs/1
  Brake Torque/1 -> Abs1/1
  Relational Operator/1 -> Logical Operator1/2, Logical Operator2/1
  Logical Operator1/1 -> SR-Memory/2(Set)
  Constant/1 -> SR-Memory/1(Signal)
  Logical Operator2/1 -> SR-Memory/3(Reset)
  SR-Memory/1(Out) -> Sum/1, Memory1/1
  Switch/1 -> ax_out/1
  Sum/1 -> Switch/2
  ax is 0/1 -> Switch/3
  Constant1/1 -> Sum/2
  v0/1 -> Product/1
  Product/1 -> x0/1
  Configurable Subsystem/1(Out1) -> Product/2
  ax/1 -> Switch/1  "ax"
  Memory1/1 -> vx_reset/1  "vx"

== system MCity_cs_withAEBSBlock/BMW_Z3_1/Dynamics_Simple/Chassis/Bicycle_model_[XYZ]/Y & Yaw_Motion/Configurable Subsystem ==
  In1 : Inport
  In2 : Inport  Port=2
  Integrator : Integrator  ExternalReset=level
  Out1 : Outport
  wires:
  In1/1 -> Integrator/1
  In2/1 -> Integrator/2
  Integrator/1 -> Out1/1

== system MCity_cs_withAEBSBlock/BMW_Z3_1/Dynamics_Simple/Chassis/Bicycle_model_[XYZ]/Y & Yaw_Motion/Configurable Subsystem1 ==
  In1 : Inport
  Integrator : Integrator
  Out1 : Outport
  wires:
  In1/1 -> Integrator/1
  Integrator/1 -> Out1/1

== system MCity_cs_withAEBSBlock/BMW_Z3_1/Dynamics_Simple/Chassis/Bicycle_model_[XYZ]/Y & Yaw_Motion/Configurable Subsystem2 ==
  In1 : Inport
  In2 : Inport  Port=2
  Integrator : Integrator  ExternalReset=level
  Out1 : Outport
  wires:
  In1/1 -> Integrator/1
  In2/1 -> Integrator/2
  Integrator/1 -> Out1/1

== system MCity_cs_withAEBSBlock/BMW_Z3_1/Dynamics_Simple/Chassis/Bicycle_model_[XYZ]/Z, Pitch_Motion & Roll_Motion/Configurable Subsystem ==
  In1 : Inport
  Integrator : Integrator  LimitOutput=on  UpperSaturationLimit=5*pi/180  LowerSaturationLimit=-5*pi/180
  Out1 : Outport
  wires:
  In1/1 -> Integrator/1
  Integrator/1 -> Out1/1

== system MCity_cs_withAEBSBlock/BMW_Z3_1/Dynamics_Simple/Chassis/Bicycle_model_[XYZ]/Z, Pitch_Motion & Roll_Motion/Configurable Subsystem1 ==
  In1 : Inport
  Integrator : Integrator
  Out1 : Outport
  wires:
  In1/1 -> Integrator/1
  Integrator/1 -> Out1/1

== system MCity_cs_withAEBSBlock/BMW_Z3_1/Dynamics_Simple/Chassis/Bicycle_model_[XYZ]/Z, Pitch_Motion & Roll_Motion/Configurable Subsystem2 ==
  In1 : Inport
  Integrator : Integrator
  Out1 : Outport
  wires:
  In1/1 -> Integrator/1
  Integrator/1 -> Out1/1

== system MCity_cs_withAEBSBlock/BMW_Z3_1/Dynamics_Simple/Chassis/Bicycle_model_[XYZ]/Z, Pitch_Motion & Roll_Motion/Configurable Subsystem3 ==
  In1 : Inport
  Integrator : Integrator
  Out1 : Outport
  wires:
  In1/1 -> Integrator/1
  Integrator/1 -> Out1/1

== system MCity_cs_withAEBSBlock/BMW_Z3_1/Dynamics_Simple/Chassis/Bicycle_model_[XYZ]/Z, Pitch_Motion & Roll_Motion/Configurable Subsystem4 ==
  In1 : Inport
  Integrator : Integrator
  Out1 : Outport
  wires:
  In1/1 -> Integrator/1
  Integrator/1 -> Out1/1

== system MCity_cs_withAEBSBlock/BMW_Z3_1/Dynamics_Simple/Chassis/Bicycle_model_[XYZ]/Z, Pitch_Motion & Roll_Motion/Configurable Subsystem5 ==
  In1 : Inport
  Integrator : Integrator
  Out1 : Outport
  wires:
  In1/1 -> Integrator/1
  Integrator/1 -> Out1/1

== system MCity_cs_withAEBSBlock/BMW_Z3_1/Dynamics_Simple/Chassis/Bicycle_model_[XYZ]/Z, Pitch_Motion & Roll_Motion/Configurable Subsystem9 ==
  In1 : Inport
  Derivative : Derivative
  Out1 : Outport
  wires:
  In1/1 -> Derivative/1
  Derivative/1 -> Out1/1

== system MCity_cs_withAEBSBlock/BMW_Z3_1/Dynamics_Simple/Chassis/FrontTyre/AlphaFront/Enabled Subsystem ==
  In : Inport
  Enable : EnablePort  PropagateVarSize=During execution
  AlphaFront : Fcn  Expr=-atan( (u(2)+u(3)*p.a)/u(1) )
  Alpha : Outport  OutputWhenDisabled=reset  InitialOutput=[0]
  wires:
  AlphaFront/1 -> Alpha/1
  In/1 -> AlphaFront/1

== system MCity_cs_withAEBSBlock/BMW_Z3_1/Dynamics_Simple/Chassis/RearTyre/AlphaRear/Enabled Subsystem ==
  In : Inport
  Enable : EnablePort  PropagateVarSize=During execution
  AlphaRear : Fcn  Expr=-atan( (u(2)-u(3)*p.b)/u(1) )
  Alpha : Outport  OutputWhenDisabled=reset  InitialOutput=[0]
  wires:
  AlphaRear/1 -> Alpha/1
  In/1 -> AlphaRear/1

== system MCity_cs_withAEBSBlock/BMW_Z3_1/Subsystem/PreBraking Model/Bend road segment/T1.6/median filter ==
  Flag in : Inport
  Memory : Memory  InheritSampleTime=on
  Memory1 : Memory  InheritSampleTime=on
  Mux : Mux  Inputs=3
  median function : MATLAB Function  TreatAsAtomicUnit=on
  Flag out : Outport
  wires:
  Flag in/1 -> Mux/1, Memory/1
  Memory/1 -> Mux/2, Memory1/1
  Memory1/1 -> Mux/3
  Mux/1 -> median function/1(u)
  median function/1(y) -> Flag out/1

== system MCity_cs_withAEBSBlock/BMW_Z3_1/Subsystem/PreBraking Model/Bend road segment/T2.6/median filter ==
  Flag in : Inport
  Memory : Memory  InheritSampleTime=on
  Memory1 : Memory  InheritSampleTime=on
  Mux : Mux  Inputs=3
  median function : MATLAB Function  TreatAsAtomicUnit=on
  Flag out : Outport
  wires:
  Flag in/1 -> Mux/1, Memory/1
  Memory/1 -> Mux/2, Memory1/1
  Memory1/1 -> Mux/3
  Mux/1 -> median function/1(u)
  median function/1(y) -> Flag out/1

== system MCity_cs_withAEBSBlock/BMW_Z3_1/Subsystem/PreBraking Model/Straight road segment/T1.6/median filter ==
  Flag in : Inport
  Memory : Memory  InheritSampleTime=on
  Memory1 : Memory  InheritSampleTime=on
  Mux : Mux  Inputs=3
  median function : MATLAB Function  TreatAsAtomicUnit=on
  Flag out : Outport
  wires:
  Flag in/1 -> Mux/1, Memory/1
  Memory/1 -> Mux/2, Memory1/1
  Memory1/1 -> Mux/3
  Mux/1 -> median function/1(u)
  median function/1(y) -> Flag out/1

== system MCity_cs_withAEBSBlock/BMW_Z3_1/Subsystem/PreBraking Model/Straight road segment/T2.6/median filter ==
  Flag in : Inport
  Memory : Memory  InheritSampleTime=on
  Memory1 : Memory  InheritSampleTime=on
  Mux : Mux  Inputs=3
  median function : MATLAB Function  TreatAsAtomicUnit=on
  Flag out : Outport
  wires:
  Flag in/1 -> Mux/1, Memory/1
  Memory/1 -> Mux/2, Memory1/1
  Memory1/1 -> Mux/3
  Mux/1 -> median function/1(u)
  median function/1(y) -> Flag out/1

== system MCity_cs_withAEBSBlock/BMW_Z3_1/Trajectories/Traj2State1/Traj2State2/Traj2MuxState_Ext/demux ==
  traj : Inport
  Demux : Demux  Outputs=18
  x : Outport
  y : Outport  Port=2
  z : Outport  Port=3
  velx : Outport  Port=4
  vely : Outport  Port=5
  velz : Outport  Port=6
  R : Outport  Port=7
  P : Outport  Port=8
  Y : Outport  Port=9
  velR : Outport  Port=10
  velP : Outport  Port=11
  velY : Outport  Port=12
  accx : Outport  Port=13
  accy : Outport  Port=14
  accz : Outport  Port=15
  accR : Outport  Port=16
  accP : Outport  Port=17
  accY : Outport  Port=18
  wires:
  Demux/18 -> accY/1
  Demux/17 -> accP/1
  Demux/16 -> accR/1
  Demux/15 -> accz/1
  Demux/14 -> accy/1
  Demux/13 -> accx/1
  Demux/12 -> velY/1
  Demux/11 -> velP/1
  Demux/10 -> velR/1
  Demux/9 -> velz/1
  Demux/8 -> vely/1
  Demux/7 -> velx/1
  Demux/6 -> Y/1
  Demux/5 -> P/1
  traj/1 -> Demux/1
  Demux/4 -> R/1
  Demux/3 -> z/1
  Demux/2 -> y/1
  Demux/1 -> x/1

== system MCity_cs_withAEBSBlock/Audi_A8_1/Dynamics_Simple/Chassis/Bicycle_model_[XYZ]/X_Motion/Max RPM and zero- velocity detection/Configurable Subsystem ==
  Step : Step  Time=0.0001  Before=1  After=0  SampleTime=0
  Out1 : Outport
  wires:
  Step/1 -> Out1/1

== system MCity_cs_withAEBSBlock/Audi_A8_1/Dynamics_Simple/Chassis/Bicycle_model_[XYZ]/X_Motion/Max RPM and zero- velocity detection/SR-Memory ==
  Signal : Inport
  Set : Inport  Port=2
  Reset : Inport  Port=3
  Constant : Constant  Value=0
  Detect Rise Positive : simulink/Logic and Bit Operations/Detect Rise Positive  vinit=0  InputProcessing=Inherited  OutDataTypeStr=uint8
  Detect Rise Positive1 : simulink/Logic and Bit Operations/Detect Rise Positive  vinit=0  InputProcessing=Inherited  OutDataTypeStr=uint8
  Manual Switch : ManualSwitch
  Manual Switch1 : ManualSwitch
  Switch : Switch  Criteria=u2 ~= 0
  Switch1 : Switch  Criteria=u2 ~= 0
  Unit Delay : UnitDelay  SampleTime=-1
  Out : Outport
  wires:
  Constant/1 -> Switch1/1
  Switch/1 -> Switch1/3
  Switch1/1 -> Unit Delay/1, Out/1
  Manual Switch1/1 -> Switch1/2
  Reset/1 -> Manual Switch1/2, Detect Rise Positive1/1
  Detect Rise Positive1/1 -> Manual Switch1/1
  Signal/1 -> Switch/1
  Unit Delay/1 -> Switch/3
  Set/1 -> Detect Rise Positive/1, Manual Switch/2
  Detect Rise Positive/1 -> Manual Switch/1
  Manual Switch/1 -> Switch/2

== system MCity_cs_withAEBSBlock/BMW_Z3_1/Dynamics_Simple/Chassis/Bicycle_model_[XYZ]/X_Motion/Max RPM and zero- velocity detection/Configurable Subsystem ==
  Step : Step  Time=0.0001  Before=1  After=0  SampleTime=0
  Out1 : Outport
  wires:
  Step/1 -> Out1/1

== system MCity_cs_withAEBSBlock/BMW_Z3_1/Dynamics_Simple/Chassis/Bicycle_model_[XYZ]/X_Motion/Max RPM and zero- velocity detection/SR-Memory ==
  Signal : Inport
  Set : Inport  Port=2
  Reset : Inport  Port=3
  Constant : Constant  Value=0
  Detect Rise Positive : simulink/Logic and Bit Operations/Detect Rise Positive  vinit=0  InputProcessing=Inherited  OutDataTypeStr=uint8
  Detect Rise Positive1 : simulink/Logic and Bit Operations/Detect Rise Positive  vinit=0  InputProcessing=Inherited  OutDataTypeStr=uint8
  Manual Switch : ManualSwitch
  Manual Switch1 : ManualSwitch
  Switch : Switch  Criteria=u2 ~= 0
  Switch1 : Switch  Criteria=u2 ~= 0
  Unit Delay : UnitDelay  SampleTime=-1
  Out : Outport
  wires:
  Constant/1 -> Switch1/1
  Switch/1 -> Switch1/3
  Switch1/1 -> Unit Delay/1, Out/1
  Manual Switch1/1 -> Switch1/2
  Reset/1 -> Manual Switch1/2, Detect Rise Positive1/1
  Detect Rise Positive1/1 -> Manual Switch1/1
  Signal/1 -> Switch/1
  Unit Delay/1 -> Switch/3
  Set/1 -> Detect Rise Positive/1, Manual Switch/2
  Detect Rise Positive/1 -> Manual Switch/1
  Manual Switch/1 -> Switch/2

== matlab function MCity_cs_withAEBSBlock/BMW_Z3_1/PathFollower_Preview_1/LateralController/CTRL REFERENCES/Calculate Lateral Error/eml_find_10k_lateral_error_points ==
  data: pvp input size=2; dist_psvehicle output size=10; TrajOffset_x_y_Y input size=3; ActorOffset_Left_Right input; p0 input size=2; PreviewDistance input size=10; Traj_x parameter; Traj_y parameter; Traj_t parameter; Traj_v parameter; RefreshCounter parameter
function dist_psvehicle  = eml_find_10k_lateral_error_points(pvp,TrajOffset_x_y_Y,ActorOffset_Left_Right,p0,PreviewDistance,Traj_x,Traj_y,Traj_t,Traj_v,RefreshCounter)

dist_psvehicle = emlfcn_find_10k_lateral_error_points(pvp,TrajOffset_x_y_Y,ActorOffset_Left_Right,p0,PreviewDistance,Traj_x,Traj_y,Traj_t,Traj_v,RefreshCounter);

% end function

== matlab function MCity_cs_withAEBSBlock/Audi_A8_1/PathFollower_Preview_1/LateralController/CTRL REFERENCES/Calculate Lateral Error/eml_find_10k_lateral_error_points ==
  data: pvp input size=2; dist_psvehicle output size=10; TrajOffset_x_y_Y input size=3; ActorOffset_Left_Right input; p0 input size=2; PreviewDistance input size=10; Traj_x parameter; Traj_y parameter; Traj_t parameter; Traj_v parameter; RefreshCounter parameter
function dist_psvehicle  = eml_find_10k_lateral_error_points(pvp,TrajOffset_x_y_Y,ActorOffset_Left_Right,p0,PreviewDistance,Traj_x,Traj_y,Traj_t,Traj_v,RefreshCounter)

dist_psvehicle = emlfcn_find_10k_lateral_error_points(pvp,TrajOffset_x_y_Y,ActorOffset_Left_Right,p0,PreviewDistance,Traj_x,Traj_y,Traj_t,Traj_v,RefreshCounter);

% end function

== matlab function MCity_cs_withAEBSBlock/BMW_Z3_1/PathFollower_Preview_1/LateralController/CTRL REFERENCES/Find Reference Point (pref0) on Trajectory closest to P0 Point (p0)/eml_find_closest_trajectory_points0 ==
  data: pvp input size=2; Actor_traj_distance output; TrajOffset_x_y_Y input size=3; ActorOffset_Left_Right input; p0 input size=3; Traj_x parameter; Traj_y parameter; Actor_traj_angle output; RefreshCounter parameter
function [Actor_traj_distance,Actor_traj_angle]  = eml_find_closest_trajectory_points0(pvp,TrajOffset_x_y_Y,ActorOffset_Left_Right,p0,Traj_x,Traj_y,RefreshCounter)

[Actor_traj_distance,Actor_traj_angle]  = emlfcn_find_closest_trajectory_points0(pvp,TrajOffset_x_y_Y,ActorOffset_Left_Right,p0,Traj_x,Traj_y,RefreshCounter);

% end function

== matlab function MCity_cs_withAEBSBlock/Audi_A8_1/PathFollower_Preview_1/LateralController/CTRL REFERENCES/Find Reference Point (pref0) on Trajectory closest to P0 Point (p0)/eml_find_closest_trajectory_points0 ==
  data: pvp input size=2; Actor_traj_distance output; TrajOffset_x_y_Y input size=3; ActorOffset_Left_Right input; p0 input size=3; Traj_x parameter; Traj_y parameter; Actor_traj_angle output; RefreshCounter parameter
function [Actor_traj_distance,Actor_traj_angle]  = eml_find_closest_trajectory_points0(pvp,TrajOffset_x_y_Y,ActorOffset_Left_Right,p0,Traj_x,Traj_y,RefreshCounter)

[Actor_traj_distance,Actor_traj_angle]  = emlfcn_find_closest_trajectory_points0(pvp,TrajOffset_x_y_Y,ActorOffset_Left_Right,p0,Traj_x,Traj_y,RefreshCounter);

% end function

== matlab function MCity_cs_withAEBSBlock/BMW_Z3_1/PathFollower_Preview_1/LateralController/Calculate delta steering error/eml_delta_steering_error ==
  data: v_x_vehicle input; v_x_vehicle_Min input; t_Preview_LatCtrl input; delta_steeringwheeltotal output; v_y_vehicle input; yawrate_vehicle input; CorneringStiffness_Tyres_Front input; CorneringStiffness_Tyres_Rear input; m_vehicle_total input; inertia_z_vehicle_total input; e_Lat input size=10; Pos_x_CoG_Vehicle input; wheelbase input; RefreshCounter parameter
function delta_steeringwheeltotal = eml_delta_steering_error(v_x_vehicle,v_x_vehicle_Min,t_Preview_LatCtrl,v_y_vehicle,yawrate_vehicle,CorneringStiffness_Tyres_Front,CorneringStiffness_Tyres_Rear,m_vehicle_total,inertia_z_vehicle_total,e_Lat,Pos_x_CoG_Vehicle,wheelbase,RefreshCounter)

delta_steeringwheeltotal = emlfcn_delta_steering_error(v_x_vehicle,v_x_vehicle_Min,t_Preview_LatCtrl,v_y_vehicle,yawrate_vehicle,CorneringStiffness_Tyres_Front,CorneringStiffness_Tyres_Rear,m_vehicle_total,inertia_z_vehicle_total,e_Lat,Pos_x_CoG_Vehicle,wheelbase,RefreshCounter);

% end function
